simulink model "ITSEmizgenj2"  (R2015a)
settings: Solver=ode45  StartTime=0.0  StopTime=10.0  RelTol=1e-3
values from neighbouring files (symbols this model uses):
  Kimiz3 = x(2)    [geneticj2.m]
  Kpmiz3 = x(1)    [geneticj2.m]
settings Model: Creator=PC  LastModifiedBy=PC

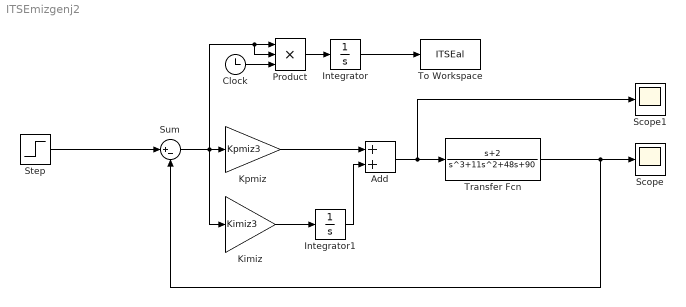
== system ITSEmizgenj2 ==
  Add : Sum
  Clock : Clock
  Integrator : Integrator
  Integrator1 : Integrator
  Kimiz : Gain  Gain=Kimiz3
  Kpmiz : Gain  Gain=Kpmiz3
  Product : Product  Inputs=3
  Scope : Scope
  Scope1 : Scope
  Step : Step  SampleTime=0
  Sum : Sum  Inputs=|+-
  To Workspace : ToWorkspace  VariableName=ITSEal  SampleTime=-1
  Transfer Fcn : TransferFcn  Numerator=[1 2]  Denominator=[1 11 48 90]
  wires:
  Sum/1 -> Product/2, Product/1, Kpmiz/1, Kimiz/1
  Step/1 -> Sum/1
  Product/1 -> Integrator/1
  Integrator/1 -> To Workspace/1
  Kimiz/1 -> Integrator1/1
  Integrator1/1 -> Add/2
  Kpmiz/1 -> Add/1
  Add/1 -> Scope1/1, Transfer Fcn/1
  Transfer Fcn/1 -> Scope/1, Sum/2
  Clock/1 -> Product/3
